simulink model "blockdemo"  (Simulink 6.3)
settings: Solver=VariableStepDiscrete  StartTime=0  StopTime=100  FixedStep=1  MaxStep=1  RelTol=1e-3
InitFcn:
  | %% DSPBuilder Start
  | alt_dspbuilder_update_model(bdroot)
  | %% DSPBuilder End
libraries: allblocks_alteradspbuilder2 x12
settings Model: Creator=mjervis  LastModifiedBy=delphick
settings OptimizationCC: BooleanDataType=off  InlineInvariantSignals=on
settings DebuggingCC: SolverPrmCheckMsg=none
settings HardwareCC: TargetUnknown=on

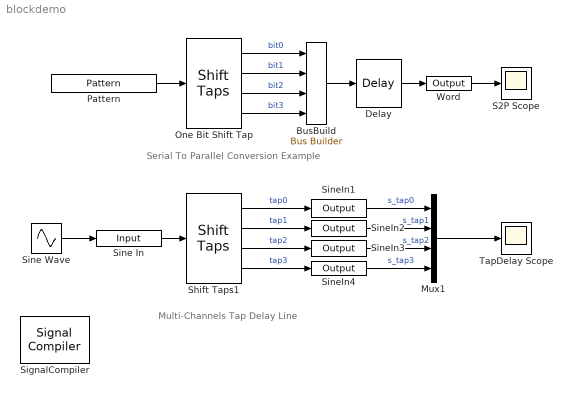
== system blockdemo ==
  note: Serial To Parallel Conversion Example
  note: Multi-Channels Tap Delay Line
  BusBuild : allblocks_alteradspbuilder2/Bus Builder  BusType=Signed Integer  bwl=4  bwr=0
  Delay : allblocks_alteradspbuilder2/Delay  pipeline=1  ClockPhase=1000  use_ena=off  use_sclr=off
  Mux1 : Mux
  One Bit Shift Tap : allblocks_alteradspbuilder2/Shift Taps  number_of_taps=4  tap_distance=1  use_shiftout=off  use_ena=off  use_sclr=off  use_dedicated_circuitry=on  ram_type=AUTO
  Pattern : allblocks_alteradspbuilder2/Pattern  Sequence=0001001000110100  SpecifyClock=off  use_ena=off  use_sclr=off
  S2P Scope : Scope
      settings: TimeRange=100  YMin=-1
  Shift Taps1 : allblocks_alteradspbuilder2/Shift Taps  number_of_taps=4  tap_distance=3  use_shiftout=off  use_ena=off  use_sclr=off  use_dedicated_circuitry=on  ram_type=AUTO
  SignalCompiler : allblocks_alteradspbuilder2/Signal Compiler  DeviceFamily=Stratix IV  DeviceName=AUTO  EnableSignalTap=off  SignalTapDepth=128  UseBoardBlock=off  StpUseDefaultClock=on  StpClock=clock
  Sine In : allblocks_alteradspbuilder2/Input  iofile=C:\workspace_clean\Documentation\DesignExamples\Tutorials\UnitBlocks\Storage\ShiftTaps\tb_blockdemo\blockdemo_Sine+In.salt  BusType=Signed Integer  bwl=8  bwr=0  SpecifyClock=off  PORTTYPE=Input
  Sine Wave : Sin  Amplitude=2^7-4  Frequency=2*pi/50  SampleTime=0
  SineIn1 : allblocks_alteradspbuilder2/Output  iofile=C:\workspace_clean\Documentation\DesignExamples\Tutorials\UnitBlocks\Storage\ShiftTaps\tb_blockdemo\blockdemo_SineIn1.capture  BusType=Signed Integer  bwl=8  bwr=0  PORTTYPE=Output
  SineIn2 : allblocks_alteradspbuilder2/Output  iofile=C:\workspace_clean\Documentation\DesignExamples\Tutorials\UnitBlocks\Storage\ShiftTaps\tb_blockdemo\blockdemo_SineIn2.capture  BusType=Signed Integer  bwl=8  bwr=0  PORTTYPE=Output
  SineIn3 : allblocks_alteradspbuilder2/Output  iofile=C:\workspace_clean\Documentation\DesignExamples\Tutorials\UnitBlocks\Storage\ShiftTaps\tb_blockdemo\blockdemo_SineIn3.capture  BusType=Signed Integer  bwl=8  bwr=0  PORTTYPE=Output
  SineIn4 : allblocks_alteradspbuilder2/Output  iofile=C:\workspace_clean\Documentation\DesignExamples\Tutorials\UnitBlocks\Storage\ShiftTaps\tb_blockdemo\blockdemo_SineIn4.capture  BusType=Signed Integer  bwl=8  bwr=0  PORTTYPE=Output
  TapDelay Scope : Scope
      settings: TimeRange=100  YMin=-150  YMax=150
  Word : allblocks_alteradspbuilder2/Output  iofile=C:\workspace_clean\Documentation\DesignExamples\Tutorials\UnitBlocks\Storage\ShiftTaps\tb_blockdemo\blockdemo_Word.capture  BusType=Signed Integer  bwl=4  bwr=0  PORTTYPE=Output
  wires:
  Pattern/1 -> One Bit Shift Tap/1
  One Bit Shift Tap/1 -> BusBuild/1  "bit0"
  One Bit Shift Tap/3 -> BusBuild/3  "bit2"
  One Bit Shift Tap/4 -> BusBuild/4  "bit3"
  Sine In/1 -> Shift Taps1/1
  Shift Taps1/1 -> SineIn1/1  "tap0"
  Shift Taps1/2 -> SineIn2/1  "tap1"
  Shift Taps1/3 -> SineIn3/1  "tap2"
  Shift Taps1/4 -> SineIn4/1  "tap3"
  Sine Wave/1 -> Sine In/1
  Mux1/1 -> TapDelay Scope/1
  One Bit Shift Tap/2 -> BusBuild/2  "bit1"
  BusBuild/1 -> Delay/1
  Delay/1 -> Word/1
  SineIn2/1 -> Mux1/2  "s_tap1"
  SineIn3/1 -> Mux1/3  "s_tap2"
  SineIn4/1 -> Mux1/4  "s_tap3"
  SineIn1/1 -> Mux1/1  "s_tap0"
  Word/1 -> S2P Scope/1
